simulink model "PID_Ctrl"  (R2020a)
settings: Solver=VariableStepAuto  StartTime=0.0  StopTime=0.2  RelTol=1e-3
PostLoadFcn:
  | J=3.2284e-6;
  | L=2.75e-6;
  | R=4;
  | Ke=0.0274;
  | Kt=0.0274;
  | b=3.5077e-6;
model workspace (MAT data in the model file):
  Kd = 0.1585
  Ki = 504.1
  Kp = 22.51
  N = 2008
settings Model: DataDictionary=DataDicn.sldd  Creator=Hp  LastModifiedBy=Hp
settings DataIOCC: SaveOutput=off  SaveTime=off

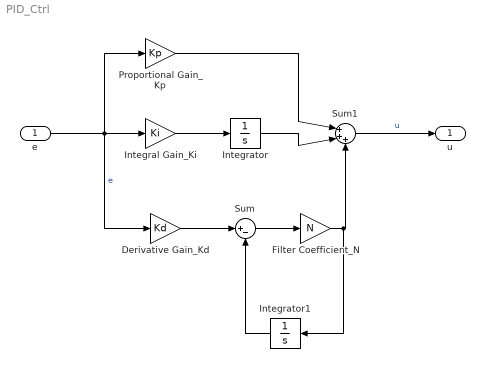
== system PID_Ctrl ==
  e : Inport  OutDataTypeStr=double  PortDimensions=1  SampleTime=0
  Derivative Gain_Kd : Gain  Gain=Kd
  Filter Coefficient_N : Gain  Gain=N
  Integral Gain_Ki : Gain  Gain=Ki
  Integrator : Integrator
  Integrator1 : Integrator
  Proportional Gain_Kp : Gain  Gain=Kp
  Sum : Sum  Inputs=|+-
  Sum1 : Sum  Inputs=|+++
  u : Outport  OutDataTypeStr=double  PortDimensions=1  SampleTime=0
  wires:
  Integrator/1 -> Sum1/2
  Integral Gain_Ki/1 -> Integrator/1
  e/1 -> Derivative Gain_Kd/1, Proportional Gain_Kp/1, Integral Gain_Ki/1  "e"
  Proportional Gain_Kp/1 -> Sum1/1
  Sum1/1 -> u/1  "u"
  Derivative Gain_Kd/1 -> Sum/1
  Sum/1 -> Filter Coefficient_N/1
  Filter Coefficient_N/1 -> Sum1/3, Integrator1/1
  Integrator1/1 -> Sum/2
